simulink model "Microgrid"  (R2025b)
settings: Solver=FixedStepAuto  StartTime=0.0  StopTime=1  FixedStep=5e-7  RelTol=1e-3
InitFcn:
  | unitlmModelFile = get_param(bdroot, 'FileName');
  | if ~isempty(unitlmModelFile), addpath(fileparts(unitlmModelFile)); end
  | initialize_unitlm_microgrid();
  | clear unitlmModelFile
StopFcn:
  | %% StopFcn: save reference-system simulation results
  | 
  | % 获取模型文件所在目录
  | modelName = bdroot;
  | modelFile = get_param(modelName, 'FileName');
  | 
  | if isempty(modelFile)
  |     % 模型尚未保存时，使用当前工作目录
  |     modelDir = pwd;
  | else
  |     modelDir = fileparts(modelFile);
  | end
  | 
  | % 创建 result 文件夹
  | resultDir = fullfile(modelDir, 'result');
  | 
  | if ~exist(resultDir, 'dir')
  |     mkdir(resultDir);
  | end
  | 
  | % 需要保存的工作区变量
  | variableNames = {
  |     'server_voltage'
  |     'server_current'
  |     'server_PQ'
  |     'client_voltage'
  |     'client_current'
  |     'client_PQ'
  |     'client_omega'
  | };
  | 
  | % 用结构体保存，并添加 _ref 后缀
  | refData = struct();
  | 
  | for k = 1:numel(variableNames)
  | 
  |     originalName = variableNames{k};
  |     refName      = [originalName, '_ref'];
  | 
  |     % 检查变量是否存在于 Base Workspace
  |     variableExists = evalin( ...
  |         'base', ...
  |         sprintf('exist(''%s'', ''var'')', originalName));
  | 
  |     if variableExists
  |         refData.(refName) = evalin('base', originalName);
  |     else
  |         warning( ...
  |             'StopFcn:MissingVariable', ...
  |             'Variable "%s" was not found in the base workspace.', ...
  |             originalName);
  |     end
  | end
  | 
  | % 保存为 result/ref_system.mat
  | saveFile = fullfile(resultDir, 'ref_system.mat');
  | save(saveFile, '-struct', 'refData');
  | 
  | fprintf('Reference-system results saved to:\n%s\n', saveFile);
values from neighbouring files (symbols this model uses):
  Cf = Cf_pu*Cb    [initialize_unitlm_microgrid.m]
  f = logspace(log10(fMin), log10(fMax), nFrequency).'    [fit_non_heaviside_line_rational.m]    (also in initialize_unitlm_microgrid.m = 50)
  fsw1 = 10e3    (= 10000)    [initialize_unitlm_microgrid.m]
  gfm_AngleKi = 3    [initialize_unitlm_microgrid.m]
  gfm_AngleKp = 1.2    [initialize_unitlm_microgrid.m]
  gfm_PrefPu = 1.0    (= 1)    [initialize_unitlm_microgrid.m]
  gfm_VloopKi = 120    [initialize_unitlm_microgrid.m]
  gfm_VloopKp = 0.08    [initialize_unitlm_microgrid.m]
  gfm_VrefPu = 0.93    [initialize_unitlm_microgrid.m]
  Ip = 2*P/(3*Vp)    [initialize_unitlm_microgrid.m]
  L1 = L1_pu*Lb    [initialize_unitlm_microgrid.m]
  L2 = L2_pu*Lb    [initialize_unitlm_microgrid.m]
  L3 = L3_pu*Lb    [initialize_unitlm_microgrid.m]
  L4 = L4_pu*Lb    [initialize_unitlm_microgrid.m]
  Lc = Lc_pu*Lb    [initialize_unitlm_microgrid.m]
  Lf2 = Lf2_pu*Lb    [initialize_unitlm_microgrid.m]
  P = 5e6    (= 5000000)    [initialize_unitlm_microgrid.m]
  R1 = R1_pu*Zb    [initialize_unitlm_microgrid.m]
  R2 = R2_pu*Zb    [initialize_unitlm_microgrid.m]
  R3 = R3_pu*Zb    [initialize_unitlm_microgrid.m]
  R4 = R4_pu*Zb    [initialize_unitlm_microgrid.m]
  Rdamp = Rf    [initialize_unitlm_microgrid.m]
  Rf = Rf_pu*Zb    [initialize_unitlm_microgrid.m]
  Rload1 = Vp/Ip    [initialize_unitlm_microgrid.m]
  Rload2 = Vp/Ip    [initialize_unitlm_microgrid.m]
  Rload3 = Vp/Ip    [initialize_unitlm_microgrid.m]
  Rv_pu = 0.1    [initialize_unitlm_microgrid.m]
  Sxfmr = 6.3e6    (= 6300000)    [initialize_unitlm_microgrid.m]
  Vac = sqrt(2)*Vline/sqrt(3)    [initialize_unitlm_microgrid.m]
  Vdc = 1350    [initialize_unitlm_microgrid.m]
  Vhv = 66e3    (= 66000)    [initialize_unitlm_microgrid.m]
  Vline = 690    [initialize_unitlm_microgrid.m]
  Vp = Vac    [initialize_unitlm_microgrid.m]
  Wb = 2*pi*f    (= 314.159265359)    [initialize_unitlm_microgrid.m]
  Xv_pu = 0.3    [initialize_unitlm_microgrid.m]
undefined symbols (not defined in the file or in its folder): DiscIntNeverNeededParam, DPL, Lline1
libraries: spsThreePhaseSeriesRLCBranchLib x17, spsControlledVoltageSourceLib x9, spsabctodq0Lib x9, spsThreePhaseVIMeasurementLib x8, slpidlib x7, spsPower3phInstantaneousLib x4, spsThreePhaseBreakerLib x4, spsThreePhaseTransformerTwoWindingsLib x4, spsdq0toabcLib x3, SimplusGT x3, spsDCVoltageSourceLib x1, spsDistributedParametersLineLib x1
(part 1 of 3)
settings Model: Creator=L  LastModifiedBy=Zhai Xinjie
settings SolverCC: AlgebraicLoopSolver=TrustRegion
settings DataIOCC: LimitDataPoints=on  SaveFormat=Array  ReturnWorkspaceOutputs=off
settings OptimizationCC: ReuseModelBlockBuffer=off  LifeSpan=inf
settings DebuggingCC: UnderspecifiedInitializationDetection=Classic  MergeDetectMultiDrivingBlocksExec=none  SolverPrmCheckMsg=warning  UnconnectedInputMsg=warning  UnconnectedOutputMsg=warning  UnconnectedLineMsg=warning  StateNameClashWarn=warning  SFUnexpectedBacktrackingDiag=warning  SFNoUnconditionalDefaultTransitionDiag=warning  SFExecutionAtInitializationDiag=none  ArithmeticOperatorsInVariantConditions=warning
settings HardwareCC: ProdBitPerPointer=32.0  ProdBitPerSizeT=32.0  ProdBitPerPtrDiffT=32.0  ProdLargestAtomicFloat=None  ProdIntDivRoundTo=Undefined  ProdEndianess=Unspecified  ProdWordSize=32.0  ProdHWDeviceType=32-bit Generic
settings ModelReferenceCC: EnableRefExpFcnMdlSchedulingChecks=on  PropagateSignalLabelsOutOfModel=off
settings SFSimCC: SimUseLocalCustomCode=off  CustomCodeUndefinedFunction=UseInterfaceOnly
settings RTWCC: RTWUseLocalCustomCode=off  GPUComputeCapability=3.5  DLArmComputeVersion=19.05
settings CodeAppCC: StateflowObjectComments=on
settings GRTTargetCC: TargetLangStandard=C89/C90 (ANSI)
settings ConfigComp: CovMetricSettings=dw  CovSaveCumulativeToWorkspaceVar=on  CovSaveSingleToWorkspaceVar=on  CovExternalEMLEnable=off
settings SimscapeCC: SimscapeNormalizeSystem=off

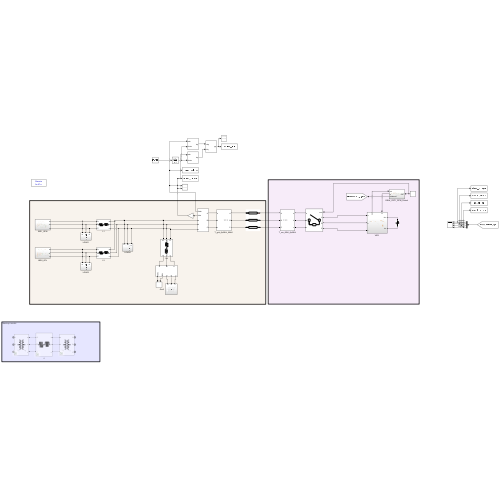
[thumbnail: Simulink's stored preview of the top-level diagram]
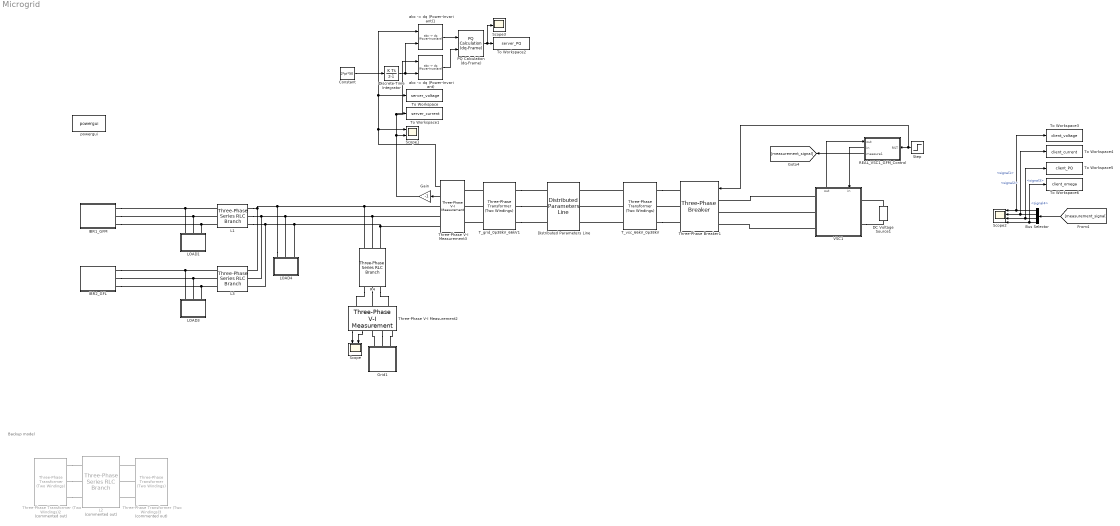
== system Microgrid ==
  note: Backup model
  Bus Selector : BusSelector  OutputSignals=signal1,signal2,signal3,signal4
  Constant : Constant  Value=2*pi*50
  DC Voltage Source1 : spsDCVoltageSourceLib/DC Voltage Source  Amplitude=Vdc  Measurements=None
  Discrete-Time Integrator : DiscreteIntegrator  SampleTime=-1  ICPrevOutput=DiscIntNeverNeededParam  ICPrevScaledInput=DiscIntNeverNeededParam
  Distributed Parameters Line : spsDistributedParametersLineLib/Distributed Parameters Line  Phases=3  Length=DPL.originalLength  Frequency=f  Resistance=DPL.R  Inductance=DPL.L  Capacitance=DPL.C  x1=[-0.0002325 0 0 0;-0.000232 0 0 0;-0.0002315 0 0 0;-0.000231 0 0 0;-0.0002305 0 0 0;-0.00023 0 0 0;-0.0002295 0 0 0;-0.000229 0 0 0;-0.0002285 0 0 0;-0.000228 0 0 0;-0.0002275 0 0 0;-0.000227 0 0 0;-0.0002265 0 0 0;-0.000226 0 0 0;-0.0002255 0 0 0;-0.000225 0 0 0;-0.0002245 0 0 0;-0.000224 0 0 0;-0.0002235 0 0 0;-0.000223 0 0 0;-0.0002225 0 0 0;-0.000222 0 0 0;-0.0002215 0 0 0;-0.000221 0 0 0;-0.0002205 0 0 0;-0.00022 0 0 0;-0.0002195 0 0 0;-0.000219 0 0 0;-0.0002185 0 0 0;-0.000218 0 0 0;-0.0002175 0 0 0;-0.000217 0 0 0;-0.0002165 0 0 0;-0.000216 0 0 0;-0.0002155 0 0 0;-0.000215 0 0 0;-0.0002145 0 0 0;-0.000214 0 0 0;-0.0002135 0 0 0;-0.000213 0 0 0;-0.0002125 0 0 0;-0.000212 0 0 0;-0.0002115 0 0 0;-0.000211 0 0 0;-0.0002105 0 0 0;-0.00021 0 0 0;-0.0002095 0 0 0;-0.000209 0 0 0;-0.0002085 0 0 0;-0.000208 0 0 0;-0.0002075 0 0 0;-0.000207 0 0 0;-0.0002065 0 0 0;-0.000206 0 0 0;-0.0002055 0 0 0;-0.000205 0 0 0;-0.0002045 0 0 0;-0.000204 0 0 0;-0.0002035 0 0 0;-0.000203 0 0 0;-0.0002025 0 0 0;-0.000202 0 0 0;-0.0002015 0 0 0;-0.000201 0 0 0;-0.0002005 0 0 0;-0.0002 0 0 0;-0.0001995 0 0 0;-0.000199 0 0 0;-0.0001985 0 0 0;-0.000198 0 0 0;-0.0001975 0 0 0;-0.000197 0 0 0;-0.0001965 0 0 0;-0.000196 0 0 0;-0.0001955 0 0 0;-0.000195 0 0 0;-0.0001945 0 0 0;-0.000194 0 0 0;-0.0001935 0 0 0;-0.000193 0 0 0;-0.0001925 0 0 0;-0.000192 0 0 0;-0.0001915 0 0 0;-0.000191 0 0 0;-0.0001905 0 0 0;-0.00019 0 0 0;-0.0001895 0 0 0;-0.000189 0 0 0;-0.0001885 0 0 0;-0.000188 0 0 0;-0.0001875 0 0 0;-0.000187 0 0 0;-0.0001865 0 0 0;-0.000186 0 0 0;-0.0001855 0 0 0;-0.000185 0 0 0;-0.0001845 0 0 0;-0.000184 0 0 0;-0.0001835 0 0 0;-0.000183 0 0 0;-0.0001825 0 0 0;-0.000182 0 0 0;-0.0001815 0 0 0;-0.000181 0 0 0;-0.0001805 0 0 0;-0.00018 0 0 0;-0.0001795 0 0 0;-0.000179 0 0 0;-0.0001785 0 0 0;-0.000178 0 0 0;-0.0001775 0 0 0;-0.000177 0 0 0;-0.0001765 0 0 0;-0.000176 0 0 0;-0.0001755 0 0 0;-0.000175 0 0 0;-0.0001745 0 0 0;-0.000174 0 0 0;-0.0001735 0 0 0;-0.000173 0 0 0;-0.0001725 0 0 0;-0.000172 0 0 0;-0.0001715 0 0 0;-0.000171 0 0 0;-0.0001705 0 0 0;-0.00017 0 0 0;-0.0001695 0 0 0;-0.000169 0 0 0;-0.0001685 0 0 0;-0.000168 0 0 0;-0.0001675 0 0 0;-0.000167 0 0 0;-0.0001665 0 0 0;-0.000166 0 0 0;-0.0001655 0 0 0;-0.000165 0 0 0;-0.0001645 0 0 0;-0.000164 0 0 0;-0.0001635 0 0 0;-0.000163 0 0 0;-0.0001625 0 0 0;-0.000162 0 0 0;-0.0001615 0 0 0;-0.000161 0 0 0;-0.0001605 0 0 0;-0.00016 0 0 0;-0.0001595 0 0 0;-0.000159 0 0 0;-0.0001585 0 0 0;-0.000158 0 0 0;-0.0001575 0 0 0;-0.000157 0 0 0;-0.0001565 0 0 0;-0.000156 0 0 0;-0.0001555 0 0 0;-0.000155 0 0 0;-0.0001545 0 0 0;-0.000154 0 0 0;-0.0001535 0 0 0;-0.000153 0 0 0;-0.0001525 0 0 0;-0.000152 0 0 0;-0.0001515 0 0 0;-0.000151 0 0 0;-0.0001505 0 0 0;-0.00015 0 0 0;-0.0001495 0 0 0;-0.000149 0 0 0;-0.0001485 0 0 0;-0.000148 0 0 0;-0.0001475 0 0 0;-0.000147 0 0 0;-0.0001465 0 0 0;-0.000146 0 0 0;-0.0001455 0 0 0;-0.000145 0 0 0;-0.0001445 0 0 0;-0.000144 0 0 0;-0.0001435 0 0 0;-0.000143 0 0 0;-0.0001425 0 0 0;-0.000142 0 0 0;-0.0001415 0 0 0;-0.000141 0 0 0;-0.0001405 0 0 0;-0.00014 0 0 0;-0.0001395 0 0 0;-0.000139 0 0 0;-0.0001385 0 0 0;-0.000138 0 0 0;-0.0001375 0 0 0;-0.000137 0 0 0;-0.0001365 0 0 0;-0.000136 0 0 0;-0.0001355 0 0 0;-0.000135 0 0 0;-0.0001345 0 0 0;-0.000134 0 0 0;-0.0001335 0 0 0;-0.000133 0 0 0;-0.0001325 0 0 0;-0.000132 0 0 0;-0.0001315 0 0 0;-0.000131 0 0 0;-0.0001305 0 0 0;-0.00013 0 0 0;-0.0001295 0 0 0;-0.000129 0 0 0;-0.0001285 0 0 0;-0.000128 0 0 0;-0.0001275 0 0 0;-0.000127 0 0 0;-0.0001265 0 0 0;-0.000126 0 0 0;-0.0001255 0 0 0;-0.000125 0 0 0;-0.0001245 0 0 0;-0.000124 0 0 0;-0.0001235 0 0 0;-0.000123 0 0 0;-0.0001225 0 0 0;-0.000122 0 0 0;-0.0001215 0 0 0;-0.000121 0 0 0;-0.0001205 0 0 0;-0.00012 0 0 0;-0.0001195 0 0 0;-0.000119 0 0 0;-0.0001185 0 0 0;-0.000118 0 0 0;-0.0001175 0 0 0;-0.000117 0 0 0;-0.0001165 0 0 0;-0.000116 0 0 0;-0.0001155 0 0 0;-0.000115 0 0 0;-0.0001145 0 0 0;-0.000114 0 0 0;-0.0001135 0 0 0;-0.000113 0 0 0;-0.0001125 0 0 0;-0.000112 0 0 0;-0.0001115 0 0 0 ...(+3413 chars)]  x2=[-0.0002325 0 0 0;-0.000232 0 0 0;-0.0002315 0 0 0;-0.000231 0 0 0;-0.0002305 0 0 0;-0.00023 0 0 0;-0.0002295 0 0 0;-0.000229 0 0 0;-0.0002285 0 0 0;-0.000228 0 0 0;-0.0002275 0 0 0;-0.000227 0 0 0;-0.0002265 0 0 0;-0.000226 0 0 0;-0.0002255 0 0 0;-0.000225 0 0 0;-0.0002245 0 0 0;-0.000224 0 0 0;-0.0002235 0 0 0;-0.000223 0 0 0;-0.0002225 0 0 0;-0.000222 0 0 0;-0.0002215 0 0 0;-0.000221 0 0 0;-0.0002205 0 0 0;-0.00022 0 0 0;-0.0002195 0 0 0;-0.000219 0 0 0;-0.0002185 0 0 0;-0.000218 0 0 0;-0.0002175 0 0 0;-0.000217 0 0 0;-0.0002165 0 0 0;-0.000216 0 0 0;-0.0002155 0 0 0;-0.000215 0 0 0;-0.0002145 0 0 0;-0.000214 0 0 0;-0.0002135 0 0 0;-0.000213 0 0 0;-0.0002125 0 0 0;-0.000212 0 0 0;-0.0002115 0 0 0;-0.000211 0 0 0;-0.0002105 0 0 0;-0.00021 0 0 0;-0.0002095 0 0 0;-0.000209 0 0 0;-0.0002085 0 0 0;-0.000208 0 0 0;-0.0002075 0 0 0;-0.000207 0 0 0;-0.0002065 0 0 0;-0.000206 0 0 0;-0.0002055 0 0 0;-0.000205 0 0 0;-0.0002045 0 0 0;-0.000204 0 0 0;-0.0002035 0 0 0;-0.000203 0 0 0;-0.0002025 0 0 0;-0.000202 0 0 0;-0.0002015 0 0 0;-0.000201 0 0 0;-0.0002005 0 0 0;-0.0002 0 0 0;-0.0001995 0 0 0;-0.000199 0 0 0;-0.0001985 0 0 0;-0.000198 0 0 0;-0.0001975 0 0 0;-0.000197 0 0 0;-0.0001965 0 0 0;-0.000196 0 0 0;-0.0001955 0 0 0;-0.000195 0 0 0;-0.0001945 0 0 0;-0.000194 0 0 0;-0.0001935 0 0 0;-0.000193 0 0 0;-0.0001925 0 0 0;-0.000192 0 0 0;-0.0001915 0 0 0;-0.000191 0 0 0;-0.0001905 0 0 0;-0.00019 0 0 0;-0.0001895 0 0 0;-0.000189 0 0 0;-0.0001885 0 0 0;-0.000188 0 0 0;-0.0001875 0 0 0;-0.000187 0 0 0;-0.0001865 0 0 0;-0.000186 0 0 0;-0.0001855 0 0 0;-0.000185 0 0 0;-0.0001845 0 0 0;-0.000184 0 0 0;-0.0001835 0 0 0;-0.000183 0 0 0;-0.0001825 0 0 0;-0.000182 0 0 0;-0.0001815 0 0 0;-0.000181 0 0 0;-0.0001805 0 0 0;-0.00018 0 0 0;-0.0001795 0 0 0;-0.000179 0 0 0;-0.0001785 0 0 0;-0.000178 0 0 0;-0.0001775 0 0 0;-0.000177 0 0 0;-0.0001765 0 0 0;-0.000176 0 0 0;-0.0001755 0 0 0;-0.000175 0 0 0;-0.0001745 0 0 0;-0.000174 0 0 0;-0.0001735 0 0 0;-0.000173 0 0 0;-0.0001725 0 0 0;-0.000172 0 0 0;-0.0001715 0 0 0;-0.000171 0 0 0;-0.0001705 0 0 0;-0.00017 0 0 0;-0.0001695 0 0 0;-0.000169 0 0 0;-0.0001685 0 0 0;-0.000168 0 0 0;-0.0001675 0 0 0;-0.000167 0 0 0;-0.0001665 0 0 0;-0.000166 0 0 0;-0.0001655 0 0 0;-0.000165 0 0 0;-0.0001645 0 0 0;-0.000164 0 0 0;-0.0001635 0 0 0;-0.000163 0 0 0;-0.0001625 0 0 0;-0.000162 0 0 0;-0.0001615 0 0 0;-0.000161 0 0 0;-0.0001605 0 0 0;-0.00016 0 0 0;-0.0001595 0 0 0;-0.000159 0 0 0;-0.0001585 0 0 0;-0.000158 0 0 0;-0.0001575 0 0 0;-0.000157 0 0 0;-0.0001565 0 0 0;-0.000156 0 0 0;-0.0001555 0 0 0;-0.000155 0 0 0;-0.0001545 0 0 0;-0.000154 0 0 0;-0.0001535 0 0 0;-0.000153 0 0 0;-0.0001525 0 0 0;-0.000152 0 0 0;-0.0001515 0 0 0;-0.000151 0 0 0;-0.0001505 0 0 0;-0.00015 0 0 0;-0.0001495 0 0 0;-0.000149 0 0 0;-0.0001485 0 0 0;-0.000148 0 0 0;-0.0001475 0 0 0;-0.000147 0 0 0;-0.0001465 0 0 0;-0.000146 0 0 0;-0.0001455 0 0 0;-0.000145 0 0 0;-0.0001445 0 0 0;-0.000144 0 0 0;-0.0001435 0 0 0;-0.000143 0 0 0;-0.0001425 0 0 0;-0.000142 0 0 0;-0.0001415 0 0 0;-0.000141 0 0 0;-0.0001405 0 0 0;-0.00014 0 0 0;-0.0001395 0 0 0;-0.000139 0 0 0;-0.0001385 0 0 0;-0.000138 0 0 0;-0.0001375 0 0 0;-0.000137 0 0 0;-0.0001365 0 0 0;-0.000136 0 0 0;-0.0001355 0 0 0;-0.000135 0 0 0;-0.0001345 0 0 0;-0.000134 0 0 0;-0.0001335 0 0 0;-0.000133 0 0 0;-0.0001325 0 0 0;-0.000132 0 0 0;-0.0001315 0 0 0;-0.000131 0 0 0;-0.0001305 0 0 0;-0.00013 0 0 0;-0.0001295 0 0 0;-0.000129 0 0 0;-0.0001285 0 0 0;-0.000128 0 0 0;-0.0001275 0 0 0;-0.000127 0 0 0;-0.0001265 0 0 0;-0.000126 0 0 0;-0.0001255 0 0 0;-0.000125 0 0 0;-0.0001245 0 0 0;-0.000124 0 0 0;-0.0001235 0 0 0;-0.000123 0 0 0;-0.0001225 0 0 0;-0.000122 0 0 0;-0.0001215 0 0 0;-0.000121 0 0 0;-0.0001205 0 0 0;-0.00012 0 0 0;-0.0001195 0 0 0;-0.000119 0 0 0;-0.0001185 0 0 0;-0.000118 0 0 0;-0.0001175 0 0 0;-0.000117 0 0 0;-0.0001165 0 0 0;-0.000116 0 0 0;-0.0001155 0 0 0;-0.000115 0 0 0;-0.0001145 0 0 0;-0.000114 0 0 0;-0.0001135 0 0 0;-0.000113 0 0 0;-0.0001125 0 0 0;-0.000112 0 0 0;-0.0001115 0 0 0 ...(+3413 chars)]  x3=[-0.0002325 0 0 0;-0.000232 0 0 0;-0.0002315 0 0 0;-0.000231 0 0 0;-0.0002305 0 0 0;-0.00023 0 0 0;-0.0002295 0 0 0;-0.000229 0 0 0;-0.0002285 0 0 0;-0.000228 0 0 0;-0.0002275 0 0 0;-0.000227 0 0 0;-0.0002265 0 0 0;-0.000226 0 0 0;-0.0002255 0 0 0;-0.000225 0 0 0;-0.0002245 0 0 0;-0.000224 0 0 0;-0.0002235 0 0 0;-0.000223 0 0 0;-0.0002225 0 0 0;-0.000222 0 0 0;-0.0002215 0 0 0;-0.000221 0 0 0;-0.0002205 0 0 0;-0.00022 0 0 0;-0.0002195 0 0 0;-0.000219 0 0 0;-0.0002185 0 0 0;-0.000218 0 0 0;-0.0002175 0 0 0;-0.000217 0 0 0;-0.0002165 0 0 0;-0.000216 0 0 0;-0.0002155 0 0 0;-0.000215 0 0 0;-0.0002145 0 0 0;-0.000214 0 0 0;-0.0002135 0 0 0;-0.000213 0 0 0;-0.0002125 0 0 0;-0.000212 0 0 0;-0.0002115 0 0 0;-0.000211 0 0 0;-0.0002105 0 0 0;-0.00021 0 0 0;-0.0002095 0 0 0;-0.000209 0 0 0;-0.0002085 0 0 0;-0.000208 0 0 0;-0.0002075 0 0 0;-0.000207 0 0 0;-0.0002065 0 0 0;-0.000206 0 0 0;-0.0002055 0 0 0;-0.000205 0 0 0;-0.0002045 0 0 0;-0.000204 0 0 0;-0.0002035 0 0 0;-0.000203 0 0 0;-0.0002025 0 0 0;-0.000202 0 0 0;-0.0002015 0 0 0;-0.000201 0 0 0;-0.0002005 0 0 0;-0.0002 0 0 0;-0.0001995 0 0 0;-0.000199 0 0 0;-0.0001985 0 0 0;-0.000198 0 0 0;-0.0001975 0 0 0;-0.000197 0 0 0;-0.0001965 0 0 0;-0.000196 0 0 0;-0.0001955 0 0 0;-0.000195 0 0 0;-0.0001945 0 0 0;-0.000194 0 0 0;-0.0001935 0 0 0;-0.000193 0 0 0;-0.0001925 0 0 0;-0.000192 0 0 0;-0.0001915 0 0 0;-0.000191 0 0 0;-0.0001905 0 0 0;-0.00019 0 0 0;-0.0001895 0 0 0;-0.000189 0 0 0;-0.0001885 0 0 0;-0.000188 0 0 0;-0.0001875 0 0 0;-0.000187 0 0 0;-0.0001865 0 0 0;-0.000186 0 0 0;-0.0001855 0 0 0;-0.000185 0 0 0;-0.0001845 0 0 0;-0.000184 0 0 0;-0.0001835 0 0 0;-0.000183 0 0 0;-0.0001825 0 0 0;-0.000182 0 0 0;-0.0001815 0 0 0;-0.000181 0 0 0;-0.0001805 0 0 0;-0.00018 0 0 0;-0.0001795 0 0 0;-0.000179 0 0 0;-0.0001785 0 0 0;-0.000178 0 0 0;-0.0001775 0 0 0;-0.000177 0 0 0;-0.0001765 0 0 0;-0.000176 0 0 0;-0.0001755 0 0 0;-0.000175 0 0 0;-0.0001745 0 0 0;-0.000174 0 0 0;-0.0001735 0 0 0;-0.000173 0 0 0;-0.0001725 0 0 0;-0.000172 0 0 0;-0.0001715 0 0 0;-0.000171 0 0 0;-0.0001705 0 0 0;-0.00017 0 0 0;-0.0001695 0 0 0;-0.000169 0 0 0;-0.0001685 0 0 0;-0.000168 0 0 0;-0.0001675 0 0 0;-0.000167 0 0 0;-0.0001665 0 0 0;-0.000166 0 0 0;-0.0001655 0 0 0;-0.000165 0 0 0;-0.0001645 0 0 0;-0.000164 0 0 0;-0.0001635 0 0 0;-0.000163 0 0 0;-0.0001625 0 0 0;-0.000162 0 0 0;-0.0001615 0 0 0;-0.000161 0 0 0;-0.0001605 0 0 0;-0.00016 0 0 0;-0.0001595 0 0 0;-0.000159 0 0 0;-0.0001585 0 0 0;-0.000158 0 0 0;-0.0001575 0 0 0;-0.000157 0 0 0;-0.0001565 0 0 0;-0.000156 0 0 0;-0.0001555 0 0 0;-0.000155 0 0 0;-0.0001545 0 0 0;-0.000154 0 0 0;-0.0001535 0 0 0;-0.000153 0 0 0;-0.0001525 0 0 0;-0.000152 0 0 0;-0.0001515 0 0 0;-0.000151 0 0 0;-0.0001505 0 0 0;-0.00015 0 0 0;-0.0001495 0 0 0;-0.000149 0 0 0;-0.0001485 0 0 0;-0.000148 0 0 0;-0.0001475 0 0 0;-0.000147 0 0 0;-0.0001465 0 0 0;-0.000146 0 0 0;-0.0001455 0 0 0;-0.000145 0 0 0;-0.0001445 0 0 0;-0.000144 0 0 0;-0.0001435 0 0 0;-0.000143 0 0 0;-0.0001425 0 0 0;-0.000142 0 0 0;-0.0001415 0 0 0;-0.000141 0 0 0;-0.0001405 0 0 0;-0.00014 0 0 0;-0.0001395 0 0 0;-0.000139 0 0 0;-0.0001385 0 0 0;-0.000138 0 0 0;-0.0001375 0 0 0;-0.000137 0 0 0;-0.0001365 0 0 0;-0.000136 0 0 0;-0.0001355 0 0 0;-0.000135 0 0 0;-0.0001345 0 0 0;-0.000134 0 0 0;-0.0001335 0 0 0;-0.000133 0 0 0;-0.0001325 0 0 0;-0.000132 0 0 0;-0.0001315 0 0 0;-0.000131 0 0 0;-0.0001305 0 0 0;-0.00013 0 0 0;-0.0001295 0 0 0;-0.000129 0 0 0;-0.0001285 0 0 0;-0.000128 0 0 0;-0.0001275 0 0 0;-0.000127 0 0 0;-0.0001265 0 0 0;-0.000126 0 0 0;-0.0001255 0 0 0;-0.000125 0 0 0;-0.0001245 0 0 0;-0.000124 0 0 0;-0.0001235 0 0 0;-0.000123 0 0 0;-0.0001225 0 0 0;-0.000122 0 0 0;-0.0001215 0 0 0;-0.000121 0 0 0;-0.0001205 0 0 0;-0.00012 0 0 0;-0.0001195 0 0 0;-0.000119 0 0 0;-0.0001185 0 0 0;-0.000118 0 0 0;-0.0001175 0 0 0;-0.000117 0 0 0;-0.0001165 0 0 0;-0.000116 0 0 0;-0.0001155 0 0 0;-0.000115 0 0 0;-0.0001145 0 0 0;-0.000114 0 0 0;-0.0001135 0 0 0;-0.000113 0 0 0;-0.0001125 0 0 0;-0.000112 0 0 0;-0.0001115 0 0 0 ...(+3413 chars)]  x4=[-0.0002325 0 0 0;-0.000232 0 0 0;-0.0002315 0 0 0;-0.000231 0 0 0;-0.0002305 0 0 0;-0.00023 0 0 0;-0.0002295 0 0 0;-0.000229 0 0 0;-0.0002285 0 0 0;-0.000228 0 0 0;-0.0002275 0 0 0;-0.000227 0 0 0;-0.0002265 0 0 0;-0.000226 0 0 0;-0.0002255 0 0 0;-0.000225 0 0 0;-0.0002245 0 0 0;-0.000224 0 0 0;-0.0002235 0 0 0;-0.000223 0 0 0;-0.0002225 0 0 0;-0.000222 0 0 0;-0.0002215 0 0 0;-0.000221 0 0 0;-0.0002205 0 0 0;-0.00022 0 0 0;-0.0002195 0 0 0;-0.000219 0 0 0;-0.0002185 0 0 0;-0.000218 0 0 0;-0.0002175 0 0 0;-0.000217 0 0 0;-0.0002165 0 0 0;-0.000216 0 0 0;-0.0002155 0 0 0;-0.000215 0 0 0;-0.0002145 0 0 0;-0.000214 0 0 0;-0.0002135 0 0 0;-0.000213 0 0 0;-0.0002125 0 0 0;-0.000212 0 0 0;-0.0002115 0 0 0;-0.000211 0 0 0;-0.0002105 0 0 0;-0.00021 0 0 0;-0.0002095 0 0 0;-0.000209 0 0 0;-0.0002085 0 0 0;-0.000208 0 0 0;-0.0002075 0 0 0;-0.000207 0 0 0;-0.0002065 0 0 0;-0.000206 0 0 0;-0.0002055 0 0 0;-0.000205 0 0 0;-0.0002045 0 0 0;-0.000204 0 0 0;-0.0002035 0 0 0;-0.000203 0 0 0;-0.0002025 0 0 0;-0.000202 0 0 0;-0.0002015 0 0 0;-0.000201 0 0 0;-0.0002005 0 0 0;-0.0002 0 0 0;-0.0001995 0 0 0;-0.000199 0 0 0;-0.0001985 0 0 0;-0.000198 0 0 0;-0.0001975 0 0 0;-0.000197 0 0 0;-0.0001965 0 0 0;-0.000196 0 0 0;-0.0001955 0 0 0;-0.000195 0 0 0;-0.0001945 0 0 0;-0.000194 0 0 0;-0.0001935 0 0 0;-0.000193 0 0 0;-0.0001925 0 0 0;-0.000192 0 0 0;-0.0001915 0 0 0;-0.000191 0 0 0;-0.0001905 0 0 0;-0.00019 0 0 0;-0.0001895 0 0 0;-0.000189 0 0 0;-0.0001885 0 0 0;-0.000188 0 0 0;-0.0001875 0 0 0;-0.000187 0 0 0;-0.0001865 0 0 0;-0.000186 0 0 0;-0.0001855 0 0 0;-0.000185 0 0 0;-0.0001845 0 0 0;-0.000184 0 0 0;-0.0001835 0 0 0;-0.000183 0 0 0;-0.0001825 0 0 0;-0.000182 0 0 0;-0.0001815 0 0 0;-0.000181 0 0 0;-0.0001805 0 0 0;-0.00018 0 0 0;-0.0001795 0 0 0;-0.000179 0 0 0;-0.0001785 0 0 0;-0.000178 0 0 0;-0.0001775 0 0 0;-0.000177 0 0 0;-0.0001765 0 0 0;-0.000176 0 0 0;-0.0001755 0 0 0;-0.000175 0 0 0;-0.0001745 0 0 0;-0.000174 0 0 0;-0.0001735 0 0 0;-0.000173 0 0 0;-0.0001725 0 0 0;-0.000172 0 0 0;-0.0001715 0 0 0;-0.000171 0 0 0;-0.0001705 0 0 0;-0.00017 0 0 0;-0.0001695 0 0 0;-0.000169 0 0 0;-0.0001685 0 0 0;-0.000168 0 0 0;-0.0001675 0 0 0;-0.000167 0 0 0;-0.0001665 0 0 0;-0.000166 0 0 0;-0.0001655 0 0 0;-0.000165 0 0 0;-0.0001645 0 0 0;-0.000164 0 0 0;-0.0001635 0 0 0;-0.000163 0 0 0;-0.0001625 0 0 0;-0.000162 0 0 0;-0.0001615 0 0 0;-0.000161 0 0 0;-0.0001605 0 0 0;-0.00016 0 0 0;-0.0001595 0 0 0;-0.000159 0 0 0;-0.0001585 0 0 0;-0.000158 0 0 0;-0.0001575 0 0 0;-0.000157 0 0 0;-0.0001565 0 0 0;-0.000156 0 0 0;-0.0001555 0 0 0;-0.000155 0 0 0;-0.0001545 0 0 0;-0.000154 0 0 0;-0.0001535 0 0 0;-0.000153 0 0 0;-0.0001525 0 0 0;-0.000152 0 0 0;-0.0001515 0 0 0;-0.000151 0 0 0;-0.0001505 0 0 0;-0.00015 0 0 0;-0.0001495 0 0 0;-0.000149 0 0 0;-0.0001485 0 0 0;-0.000148 0 0 0;-0.0001475 0 0 0;-0.000147 0 0 0;-0.0001465 0 0 0;-0.000146 0 0 0;-0.0001455 0 0 0;-0.000145 0 0 0;-0.0001445 0 0 0;-0.000144 0 0 0;-0.0001435 0 0 0;-0.000143 0 0 0;-0.0001425 0 0 0;-0.000142 0 0 0;-0.0001415 0 0 0;-0.000141 0 0 0;-0.0001405 0 0 0;-0.00014 0 0 0;-0.0001395 0 0 0;-0.000139 0 0 0;-0.0001385 0 0 0;-0.000138 0 0 0;-0.0001375 0 0 0;-0.000137 0 0 0;-0.0001365 0 0 0;-0.000136 0 0 0;-0.0001355 0 0 0;-0.000135 0 0 0;-0.0001345 0 0 0;-0.000134 0 0 0;-0.0001335 0 0 0;-0.000133 0 0 0;-0.0001325 0 0 0;-0.000132 0 0 0;-0.0001315 0 0 0;-0.000131 0 0 0;-0.0001305 0 0 0;-0.00013 0 0 0;-0.0001295 0 0 0;-0.000129 0 0 0;-0.0001285 0 0 0;-0.000128 0 0 0;-0.0001275 0 0 0;-0.000127 0 0 0;-0.0001265 0 0 0;-0.000126 0 0 0;-0.0001255 0 0 0;-0.000125 0 0 0;-0.0001245 0 0 0;-0.000124 0 0 0;-0.0001235 0 0 0;-0.000123 0 0 0;-0.0001225 0 0 0;-0.000122 0 0 0;-0.0001215 0 0 0;-0.000121 0 0 0;-0.0001205 0 0 0;-0.00012 0 0 0;-0.0001195 0 0 0;-0.000119 0 0 0;-0.0001185 0 0 0;-0.000118 0 0 0;-0.0001175 0 0 0;-0.000117 0 0 0;-0.0001165 0 0 0;-0.000116 0 0 0;-0.0001155 0 0 0;-0.000115 0 0 0;-0.0001145 0 0 0;-0.000114 0 0 0;-0.0001135 0 0 0;-0.000113 0 0 0;-0.0001125 0 0 0;-0.000112 0 0 0;-0.0001115 0 0 0 ...(+3413 chars)]  x5=0.000232379000772445  V1=ones(3,3)  V2=ones(3,3)  I1=ones(3,3)  I2=ones(3,3)  nHarmo=1  Measurements=None  Decoupling=off  VsMag0=0  VrMag0=0  VsAngle0=0  VrAngle0=0  IsMag0=0  IrMag0=0  IsAngle0=0  IrAngle0=0
      settings: LibrarySourceBlock=sps_lib/Power Grid Elements/Distributed Parameters Line
  Gain : Gain  Gain=-1
  Grid1 : Subsystem
  IBR1_GFM : Subsystem
  IBR2_GFL : Subsystem
  L1 : spsThreePhaseSeriesRLCBranchLib/Three-Phase Series RLC Branch  LConnTagsString=A|B|C  RConnTagsString=A|B|C  BranchType=RL  Resistance=R1  Inductance=L1  Capacitance=1e-6  Measurements=None
  L2 : spsThreePhaseSeriesRLCBranchLib/Three-Phase Series RLC Branch  Commented=on  LConnTagsString=A|B|C  RConnTagsString=A|B|C  BranchType=RL  Resistance=R2  Inductance=L2  Capacitance=1e-6  Measurements=None
  L3 : spsThreePhaseSeriesRLCBranchLib/Three-Phase Series RLC Branch  LConnTagsString=A|B|C  RConnTagsString=A|B|C  BranchType=RL  Resistance=R3  Inductance=L3  Capacitance=1e-6  Measurements=None
  LOAD1 : Subsystem
  LOAD3 : Subsystem
  LOAD4 : Subsystem
  PQ Calculation (dq-Frame) : SimplusGT/PQ Calculation (dq-Frame)  SystemSampleTime=-1  VariantActivationTime=update diagram  EmptyChoice=off  PassThrough=off  PassThroughVariantControl=(default)  EmptyChoiceVariantControl=(default)  AllowFlexibleInterface=on  Latency=0  AutoFrameSizeCalculation=off
      settings: SourceProductName=Simplus Grid Tool
  R4 : spsThreePhaseSeriesRLCBranchLib/Three-Phase Series RLC Branch  LConnTagsString=A|B|C  RConnTagsString=A|B|C  BranchType=RL  Resistance=R4  Inductance=L4  Capacitance=1e-6  Measurements=None
  REAL_VSC1_GFM_Control : Subsystem
      settings: PortSchema="{\"entries\":[{\"content\":{\"sides\":[{\"content\":{\"connectorIds\":[\"In1\"]},\"type\":\"ConnectorPlacement.EquallySpacedRectSide\",\"uuid\":\"8a24280a-bafa-4af5-a0f6-406aa9a59b4a\"},{\"content\":{\"connectorIds\":[\"In2\",\"Out1\",\"Out2\"],\"side\":\"RIGHT\"},\"type\":\"ConnectorPlacement.EquallySpacedRectSide\",\"uuid\":\"7d4db3bb-9035-4630-ac97-c56e5fe5f777\"},{\"content\":{\"side\":\"TOP\"},\"type\":\"ConnectorPlacement.EquallySpacedRectSide\",\"uuid\":\"cf83f05c-de7f-4d84-9d8a-6900bb43b99f\"}]},\"type\":\"ConnectorPlacement.EquallySpacedConnector\",\"uuid\":\"3f42a8c1-e25b-4642-96cc-07219abe8890\"}],\"packageUris\":[\"http://schema.mathworks.com/mf0/Connector/R2020b\"],\"version\":\"1.0\"}"
  Scope : Scope  NumInputPorts=2
      settings: ActiveDisplayYMinimum=-671.75144212722125  ActiveDisplayYMaximum=671.75144212722125
  Scope1 : Scope  NumInputPorts=2
      settings: ActiveDisplayYMinimum=-1280.217166415018  ActiveDisplayYMaximum=1280.095098127161  DataLoggingVariableName=ScopeData6
  Scope2 : Scope  NumInputPorts=4
      settings: ActiveDisplayYMinimum=-1267.5019929810605  ActiveDisplayYMaximum=1267.7610259154499
  Scope3 : Scope
      settings: ActiveDisplayYMinimum=-1.9256076228718687E+7  ActiveDisplayYMaximum=1.9298921067963473E+7  DataLoggingVariableName=ScopeData7
  Step : Step  Time=0.1  SampleTime=0
  T_grid_0p38kV_66kV1 : spsThreePhaseTransformerTwoWindingsLib/Three-Phase Transformer (Two Windings)  Winding1Connection=Yg  Winding2Connection=Yg  CoreType=Three single-phase transformers  SetSaturation=off  Hysteresis=off  DataFile='hysteresis'  SetInitialFlux=off  Measurements=None  UNITS=pu  NominalPower=[Sxfmr, f]  Winding1=[Vhv, 0.002, 0.04]  Winding2=[Vline, 0.002, 0.04]  Rm=500  Lm=500  L0=0.5  Saturation=[ 0,0 ; 0.0024,1.2 ; 1.0,1.52 ]  InitialFluxes=[ 0.8 , -0.8 , 0.7 ]  BreakLoop=off  DiscreteSolver=Trapezoidal iterative  DataType=off  TransfoNumber=1
  T_vsc_66kV_0p38kV : spsThreePhaseTransformerTwoWindingsLib/Three-Phase Transformer (Two Windings)  Winding1Connection=Yg  Winding2Connection=Yg  CoreType=Three single-phase transformers  SetSaturation=off  Hysteresis=off  DataFile='hysteresis'  SetInitialFlux=off  Measurements=None  UNITS=pu  NominalPower=[Sxfmr, f]  Winding1=[Vhv, 0.002, 0.04]  Winding2=[Vline, 0.002, 0.04]  Rm=500  Lm=500  L0=0.5  Saturation=[ 0,0 ; 0.0024,1.2 ; 1.0,1.52 ]  InitialFluxes=[ 0.8 , -0.8 , 0.7 ]  BreakLoop=off  DiscreteSolver=Trapezoidal iterative  DataType=off  TransfoNumber=1
  Three-Phase Transformer (Two Windings)2 : spsThreePhaseTransformerTwoWindingsLib/Three-Phase Transformer (Two Windings)  Commented=on  Winding1Connection=Yg  Winding2Connection=Yg  CoreType=Three single-phase transformers  SetSaturation=off  Hysteresis=off  DataFile='hysteresis'  SetInitialFlux=off  Measurements=None  UNITS=pu  NominalPower=[ 250e6 , 50 ]  Winding1=[ 380e3 , 0.002 , 0.08 ]  Winding2=[ 33e3 , 0.002 , 0.08 ]  Rm=500  Lm=500  L0=0.5  Saturation=[ 0,0 ; 0.0024,1.2 ; 1.0,1.52 ]  InitialFluxes=[ 0.8 , -0.8 , 0.7 ]  BreakLoop=off  DiscreteSolver=Trapezoidal iterative  DataType=off  TransfoNumber=1
  Three-Phase Transformer (Two Windings)3 : spsThreePhaseTransformerTwoWindingsLib/Three-Phase Transformer (Two Windings)  Commented=on  Winding1Connection=Yg  Winding2Connection=Yg  CoreType=Three single-phase transformers  SetSaturation=off  Hysteresis=off  DataFile='hysteresis'  SetInitialFlux=off  Measurements=None  UNITS=pu  NominalPower=[ 250e6 , 50 ]  Winding1=[ 33e3 , 0.002 , 0.08 ]  Winding2=[ 380 , 0.002 , 0.08 ]  Rm=500  Lm=500  L0=0.5  Saturation=[ 0,0 ; 0.0024,1.2 ; 1.0,1.52 ]  InitialFluxes=[ 0.8 , -0.8 , 0.7 ]  BreakLoop=off  DiscreteSolver=Trapezoidal iterative  DataType=off  TransfoNumber=1
  Three-Phase V-I Measurement2 : spsThreePhaseVIMeasurementLib/Three-Phase V-I Measurement  VoltageMeasurement=phase-to-phase  SetLabelV=off  LabelV=Vabc1  Vpu=off  VpuLL=off  CurrentMeasurement=yes  SetLabelI=off  LabelI=Iabc3  Ipu=off  Pbase=100e6  Vbase=500e3  OutputType=Complex  PhasorSimulation=off  PSBequivalent=0
  Three-Phase V-I Measurement3 : spsThreePhaseVIMeasurementLib/Three-Phase V-I Measurement  VoltageMeasurement=phase-to-phase  SetLabelV=off  LabelV=Vabc1  Vpu=off  VpuLL=off  CurrentMeasurement=yes  SetLabelI=off  LabelI=Iabc3  Ipu=off  Pbase=100e6  Vbase=500e3  OutputType=Complex  PhasorSimulation=off  PSBequivalent=0
  Three-Phase Breaker1 : spsThreePhaseBreakerLib/Three-Phase Breaker  InitialState=open  SwitchA=on  SwitchB=on  SwitchC=on  SwitchTimes=1.5  External=on  BreakerResistance=Rbreaker  SnubberResistance=1e6  SnubberCapacitance=inf  Measurements=None
  To Workspace : ToWorkspace  VariableName=server_voltage  SaveFormat=Timeseries  SampleTime=-1
  To Workspace1 : ToWorkspace  VariableName=server_current  SaveFormat=Timeseries  SampleTime=-1
  To Workspace2 : ToWorkspace  VariableName=server_PQ  SaveFormat=Timeseries  SampleTime=-1
  To Workspace3 : ToWorkspace  VariableName=client_voltage  SaveFormat=Timeseries  SampleTime=-1
  To Workspace4 : ToWorkspace  VariableName=client_current  SaveFormat=Timeseries  SampleTime=-1
  To Workspace5 : ToWorkspace  VariableName=client_PQ  SaveFormat=Timeseries  SampleTime=-1
  To Workspace6 : ToWorkspace  VariableName=client_omega  SaveFormat=Timeseries  SampleTime=-1
  VSC1 : Subsystem
      settings: PortSchema="{\"entries\":[{\"content\":{\"sides\":[{\"content\":{\"connectorIds\":[\"LConn1\",\"LConn2\"]},\"type\":\"ConnectorPlacement.EquallySpacedRectSide\",\"uuid\":\"f9a47b7a-7ab9-4bc4-ba6a-b9374cb03391\"},{\"content\":{\"connectorIds\":[\"RConn1\",\"RConn2\",\"RConn3\"],\"side\":\"RIGHT\"},\"type\":\"ConnectorPlacement.EquallySpacedRectSide\",\"uuid\":\"cfb0475f-9637-449c-a598-06e77c9a1f18\"},{\"content\":{\"connectorIds\":[\"In1\",\"Out1\"],\"side\":\"TOP\"},\"type\":\"ConnectorPlacement.EquallySpacedRectSide\",\"uuid\":\"93622264-4e82-4ec9-8ad8-ec19c934a5ef\"},{\"content\":{\"side\":\"HIDDEN\"},\"type\":\"ConnectorPlacement.EquallySpacedRectSide\",\"uuid\":\"56686535-bc45-40fb-9bd4-cc49f520b447\"}]},\"type\":\"ConnectorPlacement.EquallySpacedConnector\",\"uuid\":\"6064451f-78f0-465c-b58b-22fa19e3979e\"}],\"packageUris\":[\"http://schema.mathworks.com/mf0/Connector/R2020b\"],\"version\":\"1.0\"}"
  "abc -> dq (Power-Invariant)" : SimplusGT/abc -> dq (Power-Invariant)  SystemSampleTime=-1  VariantActivationTime=update diagram  EmptyChoice=off  PassThrough=off  PassThroughVariantControl=(default)  EmptyChoiceVariantControl=(default)  AllowFlexibleInterface=on  Latency=0  AutoFrameSizeCalculation=off
      settings: SourceProductName=Simplus Grid Tool
  "abc -> dq (Power-Invariant)1" : SimplusGT/abc -> dq (Power-Invariant)  SystemSampleTime=-1  VariantActivationTime=update diagram  EmptyChoice=off  PassThrough=off  PassThroughVariantControl=(default)  EmptyChoiceVariantControl=(default)  AllowFlexibleInterface=on  Latency=0  AutoFrameSizeCalculation=off
      settings: SourceProductName=Simplus Grid Tool
  powergui : spspowerguiLib/powergui  Priority=1  SimulationMode=Discrete  SampleTime=5e-7  frequency=60  Iterations=50  frequencyindice=0  Pbase=100e6  ErrMax=1e-4  UnitsV=kV  UnitsW=MW  buscounter=0  FunctionMessages=off  echomessages=off  EnableUseOfTLC=off  CurrentSourceSwitches=off  DisableSnubberDevices=off  DisableRonSwitches=off  DisableVfSwitches=off  DisplayEquations=off  AutomaticDiscreteSolvers=off  SolverType=Tustin/Backward Euler (TBE)  Interpol=off  ExternalGateDelay=off  methode=off  Ts=100  x0status=blocks  SPID=on  SwTol=0  HookPort=off  NonlinearTolerance=1e-4  nMaxIteration=100  ContinueOnMaxIteration=off  RestoreLinks=warning  ResistiveCurrentMeasurement=off  Frange=[0:2:500]  Ylog=off  Xlog=on  ShowGrid=off  save=off  variable=ZData  structure=0  ZoomFFT=off  StartTime=0.0  cycles=1  DisplayStyle=1  fundamental=60  FreqAxis=off  MaxFrequency=1000  frequencyindicesteady=1  RmsSteady=1  display=off
  wires:
  REAL_VSC1_GFM_Control/1(in) -> VSC1/1(in)
  Three-Phase V-I Measurement2/1 -> Scope/1
  Three-Phase V-I Measurement2/2 -> Scope/2
  Bus Selector/1 -> To Workspace3/1, Scope2/1  "<signal1>"
  Bus Selector/2 -> To Workspace4/1, Scope2/2  "<signal2>"
  Bus Selector/3 -> To Workspace5/1, Scope2/3  "<signal3>"
  Bus Selector/4 -> To Workspace6/1, Scope2/4  "<signal4>"
  VSC1/1(out) -> REAL_VSC1_GFM_Control/2(out)
  Step/1 -> REAL_VSC1_GFM_Control/1(RST), Three-Phase Breaker1/1
  Constant/1 -> Discrete-Time Integrator/1
  Discrete-Time Integrator/1 -> "abc -> dq (Power-Invariant)"/2, "abc -> dq (Power-Invariant)1"/2
  Three-Phase V-I Measurement3/1 -> Scope1/1, To Workspace/1, "abc -> dq (Power-Invariant)1"/1
  "abc -> dq (Power-Invariant)"/1 -> PQ Calculation (dq-Frame)/2
  "abc -> dq (Power-Invariant)1"/1 -> PQ Calculation (dq-Frame)/1
  PQ Calculation (dq-Frame)/1 -> To Workspace2/1, Scope3/1
  [measurement_signal] -> Bus Selector/1
  REAL_VSC1_GFM_Control/2(measure1) -> [measurement_signal]
  Three-Phase V-I Measurement3/2 -> Gain/1
  Gain/1 -> Scope1/2, "abc -> dq (Power-Invariant)"/1, To Workspace1/1
  connections:
  LOAD4/LConn1 -- R4/LConn1 -- Three-Phase V-I Measurement3/RConn1 -- L1/RConn1 -- L3/RConn1
  LOAD3/LConn1 -- IBR2_GFL/RConn1 -- L3/LConn1
  LOAD4/LConn2 -- R4/LConn2 -- Three-Phase V-I Measurement3/RConn2 -- L1/RConn2 -- L3/RConn2
  IBR2_GFL/RConn3 -- LOAD3/LConn3 -- L3/LConn3
  IBR2_GFL/RConn2 -- LOAD3/LConn2 -- L3/LConn2
  LOAD4/LConn3 -- R4/LConn3 -- Three-Phase V-I Measurement3/RConn3 -- L1/RConn3 -- L3/RConn3
  IBR1_GFM/RConn3 -- L1/LConn3 -- LOAD1/LConn3
  L1/LConn1 -- IBR1_GFM/RConn1 -- LOAD1/LConn1
  IBR1_GFM/RConn2 -- L1/LConn2 -- LOAD1/LConn2
  Grid1/LConn1 -- Three-Phase V-I Measurement2/RConn1
  Three-Phase V-I Measurement2/RConn2 -- Grid1/LConn2
  Three-Phase V-I Measurement2/RConn3 -- Grid1/LConn3
  DC Voltage Source1/RConn1 -- VSC1/LConn1
  VSC1/LConn2 -- DC Voltage Source1/LConn1
  Three-Phase Transformer (Two Windings)3/RConn1 -- L2/RConn1
  Three-Phase Transformer (Two Windings)3/RConn2 -- L2/RConn2
  Three-Phase Transformer (Two Windings)3/RConn3 -- L2/RConn3
  Three-Phase Transformer (Two Windings)2/RConn1 -- L2/LConn1
  Three-Phase Transformer (Two Windings)2/RConn2 -- L2/LConn2
  Three-Phase Transformer (Two Windings)2/RConn3 -- L2/LConn3
  R4/RConn1 -- Three-Phase V-I Measurement2/LConn1
  R4/RConn2 -- Three-Phase V-I Measurement2/LConn2
  R4/RConn3 -- Three-Phase V-I Measurement2/LConn3
  T_grid_0p38kV_66kV1/LConn1 -- Distributed Parameters Line/RConn1
  T_grid_0p38kV_66kV1/LConn2 -- Distributed Parameters Line/RConn2
  T_grid_0p38kV_66kV1/LConn3 -- Distributed Parameters Line/RConn3
  T_grid_0p38kV_66kV1/RConn1 -- Three-Phase V-I Measurement3/LConn1
  T_grid_0p38kV_66kV1/RConn2 -- Three-Phase V-I Measurement3/LConn2
  T_grid_0p38kV_66kV1/RConn3 -- Three-Phase V-I Measurement3/LConn3
  T_vsc_66kV_0p38kV/LConn1 -- Distributed Parameters Line/LConn1
  T_vsc_66kV_0p38kV/LConn2 -- Distributed Parameters Line/LConn2
  T_vsc_66kV_0p38kV/LConn3 -- Distributed Parameters Line/LConn3
  Three-Phase Breaker1/RConn2 -- T_vsc_66kV_0p38kV/RConn2
  T_vsc_66kV_0p38kV/RConn1 -- Three-Phase Breaker1/RConn1
  T_vsc_66kV_0p38kV/RConn3 -- Three-Phase Breaker1/RConn3
  VSC1/RConn1 -- Three-Phase Breaker1/LConn1
  VSC1/RConn2 -- Three-Phase Breaker1/LConn2
  VSC1/RConn3 -- Three-Phase Breaker1/LConn3
